simulink model "verif_rocketmodel"  (R2023a)
settings: Solver=VariableStepAuto  StartTime=0.0  StopTime=60  RelTol=1e-4
values from neighbouring files (symbols this model uses):
  A2 = [0  0; 1  0]    [ss_model_altitude.mat]
  B2 = [1 0]    [ss_model_altitude.mat]
  C2 = [0 1.82012167564e-06]    [ss_model_altitude.mat]
  D2 = 0    [ss_model_altitude.mat]
  g = 9.8    [main_rocketmodel.m]    (also in main_sim_rocket.m; rocket_model.m; sim_lin.m; test_bangbang.m)
  J_T = 40267    [main_rocketmodel.m]    (also in main_sim_rocket.m; rocket_model.m = 10)
  K_z = tf(lqg_ss)    [rocket_controllerdesign_z.m]
  m = 549054    [main_rocketmodel.m]    (also in main_sim_rocket.m; rocket_model.m = 25.4; sim_lin.m; test_bangbang.m)
  sys = ss(A,B,C,D)    [controller_design.m]    (also in main_yp_fminunc.m; rocket_controllerdesign.m; rocket_controllerdesign_z.m; rocket_model.m)
  t_on = 14.6    [main_rocketmodel.m]    (also in main_sim_rocket.m; test_bangbang.m)
  Ts = 0.001    [main_rocketmodel.m]    (also in main_sim_rocket.m; sim_lin.m; square_sig.m; sum_squares_sig.m)
  x_0 = 0    [main_rocketmodel.m]    (also in main_sim_rocket.m)
  z_0 = 4000    [main_rocketmodel.m]    (also in main_sim_rocket.m; sim_lin.m; test_bangbang.m)
undefined symbols (not defined in the file or in its folder): P2
libraries: simulink x2
settings Model: Creator=bia  LastModifiedBy=bia
settings SolverCC: AlgebraicLoopSolver=TrustRegion
settings DataIOCC: ExternalInput=[t, Fe]
settings DebuggingCC: UnconnectedInputMsg=warning  UnconnectedOutputMsg=warning  UnconnectedLineMsg=warning
settings ModelReferenceCC: EnableRefExpFcnMdlSchedulingChecks=on

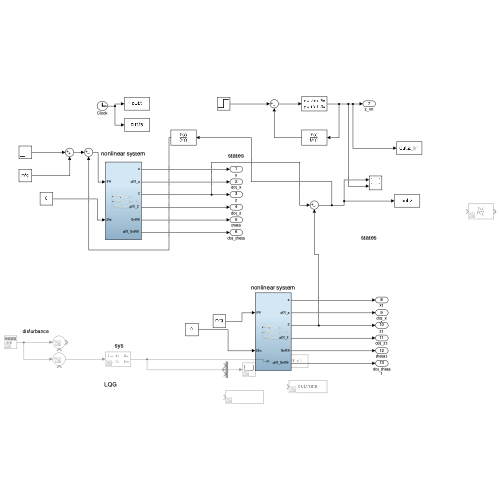
[thumbnail: Simulink's stored preview of the top-level diagram]
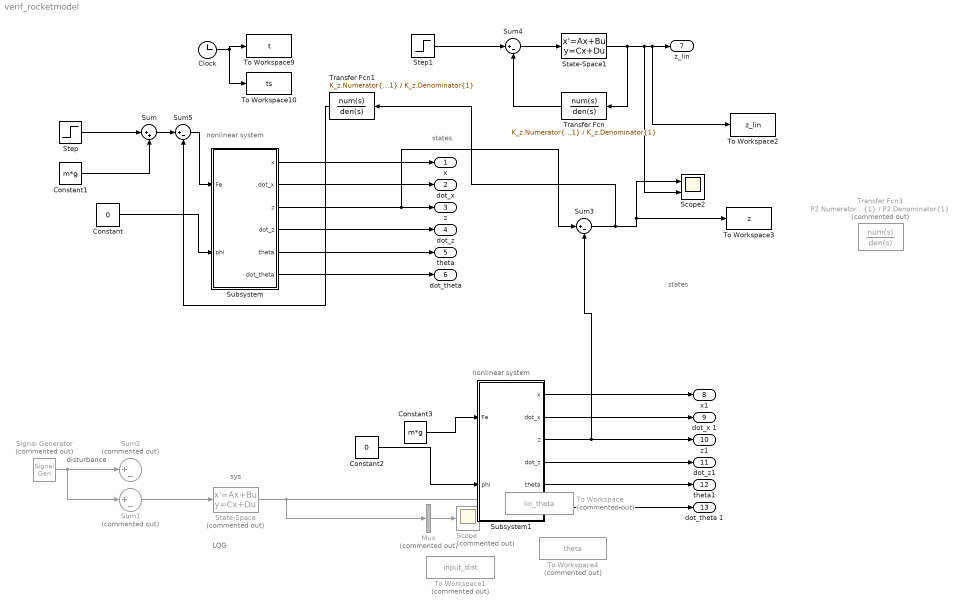
== system verif_rocketmodel ==
  note: disturbance
  note: states
  note: nonlinear system
  note: sys
  note: LQG
  note: nonlinear system
  note: states
  Clock : Clock
  Constant : Constant  Value=0
  Constant1 : Constant  Value=m*g
  Constant2 : Constant  Value=0
  Constant3 : Constant  Value=m*g
  Mux : Mux  Commented=on  Inputs=3
  Scope : Scope  Commented=on
  Scope2 : Scope  NumInputPorts=2
  Signal Generator : SignalGenerator  Commented=on  WaveForm=square  Amplitude=1e-6  Units=rad/sec
  State-Space : StateSpace  Commented=on  A=sys.A  B=sys.B  C=sys.C  D=sys.D  InitialCondition=0
  State-Space1 : StateSpace  A=A2  B=B2  C=C2  D=D2  InitialCondition=0
  Step : Step  Time=t_on  Before=0.05*7e6  After=7e6  SampleTime=0
  Step1 : Step  Time=t_on  Before=0.05*7e6  After=7e6  SampleTime=0
  Subsystem : Subsystem
  Subsystem1 : Subsystem
  Sum : Sum  Inputs=|++
  Sum1 : Sum  Commented=on  Inputs=|+-
  Sum2 : Sum  Commented=on  Inputs=|+-
  Sum3 : Sum  Inputs=|+-
  Sum4 : Sum  Inputs=|+-
  Sum5 : Sum  Inputs=|+-
  To Workspace : ToWorkspace  Commented=on  VariableName=lin_theta  SampleTime=Ts
  To Workspace1 : ToWorkspace  Commented=on  VariableName=input_dist  SampleTime=Ts
  To Workspace10 : ToWorkspace  VariableName=ts  SampleTime=Ts
  To Workspace2 : ToWorkspace  VariableName=z_lin  SampleTime=Ts
  To Workspace3 : ToWorkspace  VariableName=z  SampleTime=Ts
  To Workspace4 : ToWorkspace  Commented=on  VariableName=theta  SampleTime=Ts
  To Workspace9 : ToWorkspace  VariableName=t  SampleTime=-1
  Transfer Fcn : TransferFcn  Numerator=K_z.Numerator{1}  Denominator=K_z.Denominator{1}
  Transfer Fcn1 : TransferFcn  Numerator=K_z.Numerator{1}  Denominator=K_z.Denominator{1}
  Transfer Fcn3 : TransferFcn  Commented=on  Numerator=P2.Numerator{1}  Denominator=P2.Denominator{1}
  x : Outport
  "dot_x " : Outport  Port=2
  z : Outport  Port=3
  dot_z : Outport  Port=4
  theta : Outport  Port=5
  "dot_theta " : Outport  Port=6
  z_lin : Outport  Port=7
  x1 : Outport  Port=8
  dot_x 1 : Outport  Port=9
  z1 : Outport  Port=10
  dot_z1 : Outport  Port=11
  theta1 : Outport  Port=12
  dot_theta 1 : Outport  Port=13
  wires:
  Subsystem/5(theta) -> theta/1
  Signal Generator/1 -> Sum1/1, Sum2/1
  Subsystem/4("dot_z ") -> dot_z/1
  Subsystem/6("dot_theta ") -> "dot_theta "/1
  Subsystem/1(x) -> x/1
  Subsystem/3(z) -> Sum3/1, z/1
  Subsystem/2(dot_x) -> "dot_x "/1
  State-Space/1 -> Mux/2, To Workspace/1
  Mux/1 -> Scope/1
  Sum1/1 -> State-Space/1
  Constant/1 -> Subsystem/2(phi)
  State-Space1/1 -> Transfer Fcn/1, Scope2/2, To Workspace2/1, z_lin/1
  Constant1/1 -> Sum/2
  Subsystem1/6("dot_theta ") -> dot_theta 1/1
  Subsystem1/4("dot_z ") -> dot_z1/1
  Subsystem1/1(x) -> x1/1
  Subsystem1/5(theta) -> theta1/1
  Subsystem1/2(dot_x) -> dot_x 1/1
  Constant2/1 -> Subsystem1/2(phi)
  Subsystem1/3(z) -> z1/1, Sum3/2
  Sum3/1 -> Transfer Fcn1/1, To Workspace3/1, Scope2/1
  Step/1 -> Sum/1
  Transfer Fcn/1 -> Sum4/2
  Transfer Fcn1/1 -> Sum5/2
  Sum5/1 -> Subsystem/1(Fe)
  Sum4/1 -> State-Space1/1
  Clock/1 -> To Workspace9/1, To Workspace10/1
  Constant3/1 -> Subsystem1/1(Fe)
  Sum/1 -> Sum5/1
  Step1/1 -> Sum4/1

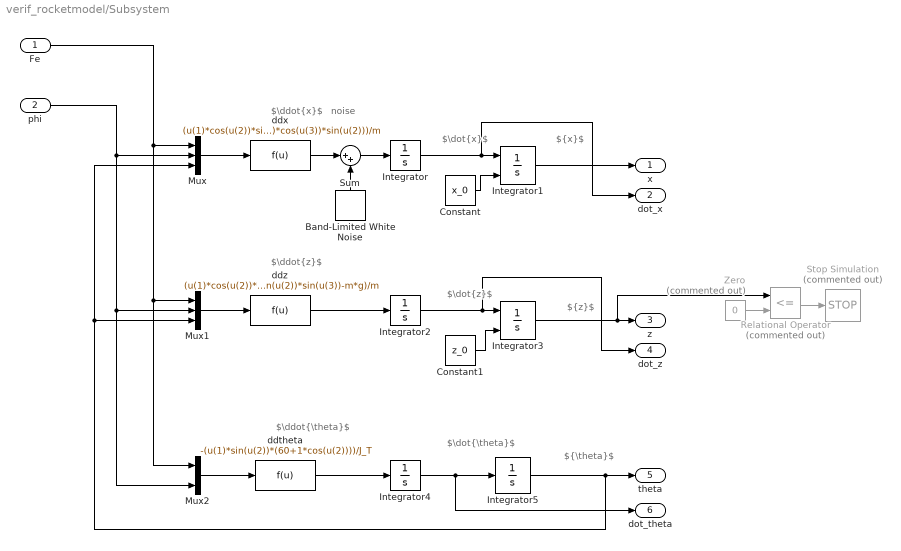
== system verif_rocketmodel/Subsystem ==
  note: $\dot{z}$
  note: $\ddot{z}$
  note: ${z}$
  note: $\ddot{\theta}$
  note: $\ddot{x}$
  note: $\dot{x}$
  note: $\dot{\theta}$
  note: ${x}$
  note: ${\theta}$
  note: noise
  Fe : Inport
  phi : Inport  Port=2
  Band-Limited White Noise : simulink/Sources/Band-Limited White Noise  Cov=0  Ts=0.1  seed=[23341]
  Constant : Constant  Value=x_0  SampleTime=Ts
  Constant1 : Constant  Value=z_0  SampleTime=Ts
  Integrator : Integrator  ContinuousStateAttributes='x_dot'
  Integrator1 : Integrator  InitialConditionSource=external  ContinuousStateAttributes='x'
  Integrator2 : Integrator  ContinuousStateAttributes='z_dot'
  Integrator3 : Integrator  InitialConditionSource=external  InitialCondition=50  LimitOutput=on  LowerSaturationLimit=0  ContinuousStateAttributes='z'
  Integrator4 : Integrator  ContinuousStateAttributes='theta_dot'
  Integrator5 : Integrator
  Mux : Mux  Inputs=3
  Mux1 : Mux  Inputs=3
  Mux2 : Mux  Inputs=2
  Relational Operator : RelationalOperator  Commented=on  Operator=<=  OutDataTypeStr=boolean  InputSameDT=off
  Stop Simulation : Stop  Commented=on
  Sum : Sum  Inputs=|++
  Zero : Constant  Commented=on  Value=0  OutDataTypeStr=Inherit: Inherit via back propagation
  ddtheta : Fcn  Expr=-(u(1)*sin(u(2))*(60+1*cos(u(2))))/J_T
  ddx : Fcn  Expr=(u(1)*cos(u(2))*sin(u(3))+u(1)*cos(u(3))*sin(u(2)))/m
  ddz : Fcn  Expr=(u(1)*cos(u(2))*cos(u(3))-u(1)*sin(u(2))*sin(u(3))-m*g)/m
  x : Outport
  dot_x : Outport  Port=2
  z : Outport  Port=3
  "dot_z " : Outport  Port=4
  theta : Outport  Port=5
  "dot_theta " : Outport  Port=6
  wires:
  ddtheta/1 -> Integrator4/1
  Mux/1 -> ddx/1
  Integrator2/1 -> "dot_z "/1, Integrator3/1
  Mux2/1 -> ddtheta/1
  Fe/1 -> Mux2/1, Mux1/1, Mux/1
  Mux1/1 -> ddz/1
  Integrator/1 -> dot_x/1, Integrator1/1
  phi/1 -> Mux2/2, Mux1/2, Mux/2
  Integrator3/1 -> z/1, Relational Operator/1
  Integrator5/1 -> Mux1/3, Mux/3, theta/1
  Constant1/1 -> Integrator3/2
  Constant/1 -> Integrator1/2
  Integrator4/1 -> Integrator5/1, "dot_theta "/1
  Zero/1 -> Relational Operator/2
  Relational Operator/1 -> Stop Simulation/1
  ddz/1 -> Integrator2/1
  Integrator1/1 -> x/1
  Band-Limited White Noise/1 -> Sum/2
  Sum/1 -> Integrator/1
  ddx/1 -> Sum/1

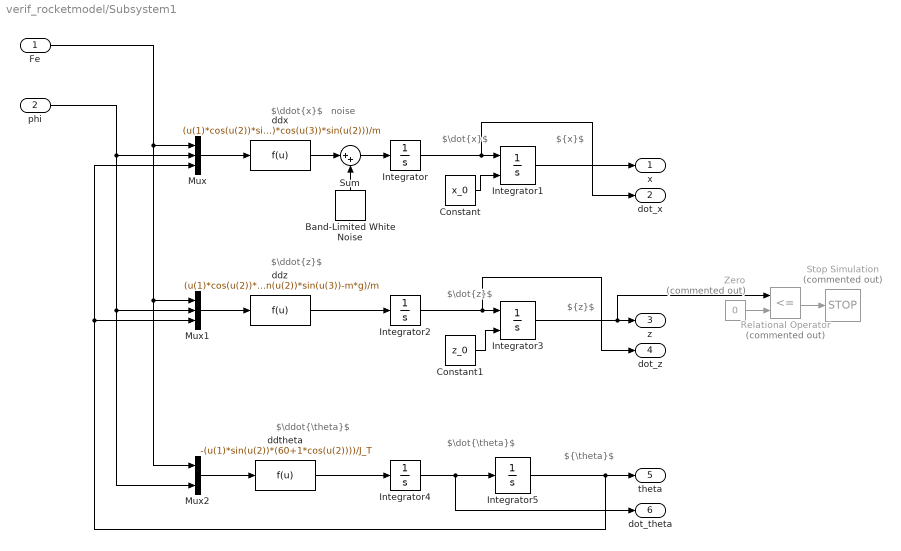
== system verif_rocketmodel/Subsystem1 ==
  note: $\dot{z}$
  note: $\ddot{z}$
  note: ${z}$
  note: $\ddot{\theta}$
  note: $\ddot{x}$
  note: $\dot{x}$
  note: $\dot{\theta}$
  note: ${x}$
  note: ${\theta}$
  note: noise
  Fe : Inport
  phi : Inport  Port=2
  Band-Limited White Noise : simulink/Sources/Band-Limited White Noise  Cov=0  Ts=0.1  seed=[23341]
  Constant : Constant  Value=x_0  SampleTime=Ts
  Constant1 : Constant  Value=z_0  SampleTime=Ts
  Integrator : Integrator  ContinuousStateAttributes='x_dot'
  Integrator1 : Integrator  InitialConditionSource=external  ContinuousStateAttributes='x'
  Integrator2 : Integrator  ContinuousStateAttributes='z_dot'
  Integrator3 : Integrator  InitialConditionSource=external  InitialCondition=50  LimitOutput=on  LowerSaturationLimit=0  ContinuousStateAttributes='z'
  Integrator4 : Integrator  ContinuousStateAttributes='theta_dot'
  Integrator5 : Integrator
  Mux : Mux  Inputs=3
  Mux1 : Mux  Inputs=3
  Mux2 : Mux  Inputs=2
  Relational Operator : RelationalOperator  Commented=on  Operator=<=  OutDataTypeStr=boolean  InputSameDT=off
  Stop Simulation : Stop  Commented=on
  Sum : Sum  Inputs=|++
  Zero : Constant  Commented=on  Value=0  OutDataTypeStr=Inherit: Inherit via back propagation
  ddtheta : Fcn  Expr=-(u(1)*sin(u(2))*(60+1*cos(u(2))))/J_T
  ddx : Fcn  Expr=(u(1)*cos(u(2))*sin(u(3))+u(1)*cos(u(3))*sin(u(2)))/m
  ddz : Fcn  Expr=(u(1)*cos(u(2))*cos(u(3))-u(1)*sin(u(2))*sin(u(3))-m*g)/m
  x : Outport
  dot_x : Outport  Port=2
  z : Outport  Port=3
  "dot_z " : Outport  Port=4
  theta : Outport  Port=5
  "dot_theta " : Outport  Port=6
  wires:
  ddtheta/1 -> Integrator4/1
  Mux/1 -> ddx/1
  Integrator2/1 -> "dot_z "/1, Integrator3/1
  Mux2/1 -> ddtheta/1
  Fe/1 -> Mux2/1, Mux1/1, Mux/1
  Mux1/1 -> ddz/1
  Integrator/1 -> dot_x/1, Integrator1/1
  phi/1 -> Mux2/2, Mux1/2, Mux/2
  Integrator3/1 -> z/1, Relational Operator/1
  Integrator5/1 -> Mux1/3, Mux/3, theta/1
  Constant1/1 -> Integrator3/2
  Constant/1 -> Integrator1/2
  Integrator4/1 -> Integrator5/1, "dot_theta "/1
  Zero/1 -> Relational Operator/2
  Relational Operator/1 -> Stop Simulation/1
  ddz/1 -> Integrator2/1
  Integrator1/1 -> x/1
  Band-Limited White Noise/1 -> Sum/2
  Sum/1 -> Integrator/1
  ddx/1 -> Sum/1
